simulink model "Circuito"  (R2014a)
settings: Solver=ode45  StartTime=0.0  StopTime=100  RelTol=1e-3
PreLoadFcn:
  | variables
InitFcn:
  | eval('variables');
  | variables
StartFcn:
  | variables
libraries: fl_lib x44, nesl_utility x5
settings Model: Creator=jhoan  LastModifiedBy=jhoan

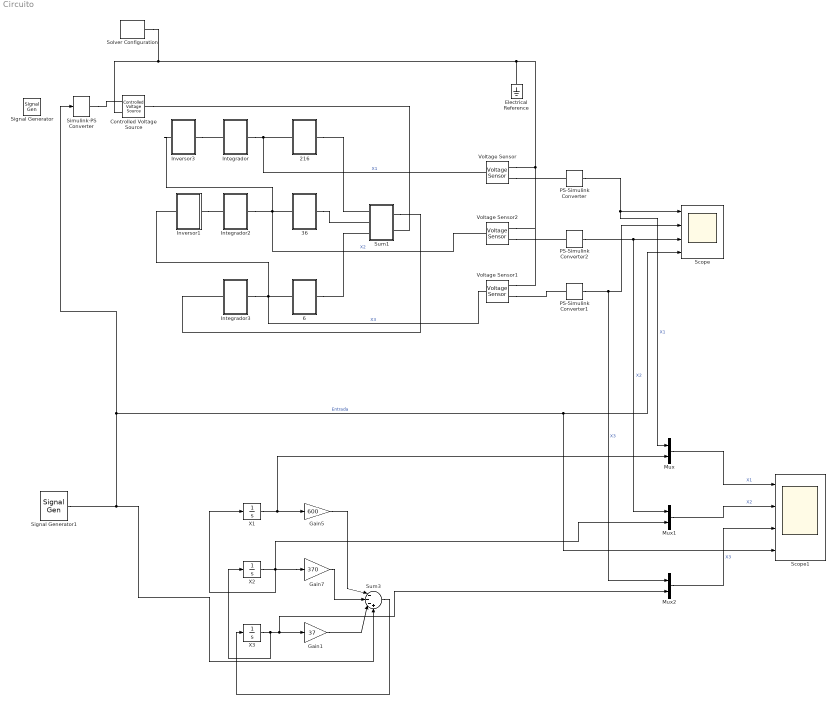
== system Circuito ==
  216 : Subsystem
  36 : Subsystem
  6 : Subsystem
  Controlled Voltage Source : fl_lib/Electrical/Electrical Sources/Controlled Voltage Source
  Electrical Reference : fl_lib/Electrical/Electrical Elements/Electrical Reference
  Gain1 : Gain  Gain=37
  Gain5 : Gain  Gain=600
  Gain7 : Gain  Gain=370
  Integrador : Subsystem
  Integrador2 : Subsystem
  Integrador3 : Subsystem
  Inversor1 : Subsystem
  Inversor3 : Subsystem
  Mux : Mux  Inputs=2
  Mux1 : Mux  Inputs=2
  Mux2 : Mux  Inputs=2
  PS-Simulink Converter : nesl_utility/PS-Simulink Converter  PhysicalDomain=network_engine_domain  SubClassName=ps_output  LeftPortType=input  RightPortType=output  PseudoPeriodic=off  Frequencies=[]  Unit=1  AffineConversion=off
  PS-Simulink Converter1 : nesl_utility/PS-Simulink Converter  PhysicalDomain=network_engine_domain  SubClassName=ps_output  LeftPortType=input  RightPortType=output  PseudoPeriodic=off  Frequencies=[]  Unit=1  AffineConversion=off
  PS-Simulink Converter2 : nesl_utility/PS-Simulink Converter  PhysicalDomain=network_engine_domain  SubClassName=ps_output  LeftPortType=input  RightPortType=output  PseudoPeriodic=off  Frequencies=[]  Unit=1  AffineConversion=off
  Scope : Scope  NumInputPorts=4
      settings: YMin=-5~-5~-5~-5  YMax=5~5~5~5
  Scope1 : Scope  NumInputPorts=4
      settings: TimeRange=0.323900041697037  YMin=-5~-5~0.09553514947454364~-5  YMax=5~5~0.09836343230282654~5  SaveName=subSimulink
  Signal Generator : SignalGenerator  Amplitude=2  Frequency=10
  Signal Generator1 : SignalGenerator  WaveForm=square  Amplitude=2  Frequency=0.1
  Simulink-PS Converter : nesl_utility/Simulink-PS Converter  PhysicalDomain=network_engine_domain  SubClassName=ps_input  LeftPortType=input  RightPortType=output  PseudoPeriodic=off  Frequencies=[]  NoiseDistribution=none  NoiseParameters=[]  Unit=1  AffineConversion=off  InputFiltering=off  SimscapeFilterOrder=1  InputFilterTimeConstant=0.001  UdotUserProvided=1
  Solver Configuration : nesl_utility/Solver Configuration  PhysicalDomain=network_engine_domain  SubClassName=solver  LeftPortType=input  RightPortType=generic  Accelerate=off  Tones=[]  Harmonics=[]  SimulateNoise=off  Profile=off  UseLocalSampling=off  EnableSwitchedLinearOptims=on  FrequencyDomain=off  UseCCode=off  RelTol=0.001  AbsTol=1e-06  MinStep=1e-09  ToWorkspace=off  DoDC=off  ResidualTolerance=1e-09  UseLocalSolver=off  LocalSolverChoice=NE_BACKWARD_EULER_ADVANCER  LocalSolverSampleTime=0.001  DoFixedCost=off  MaxNonlinIter=3  MaxModeIter=2  LinearAlgebra=Sparse  DelaysMemoryBudget=1024  AutomaticFiltering=on  FilteringTimeConstant=0.001
  Sum1 : Subsystem
  Sum3 : Sum  Inputs=|---+
  Voltage Sensor : fl_lib/Electrical/Electrical Sensors/Voltage Sensor
  Voltage Sensor1 : fl_lib/Electrical/Electrical Sensors/Voltage Sensor
  Voltage Sensor2 : fl_lib/Electrical/Electrical Sensors/Voltage Sensor
  X1 : Integrator
  X2 : Integrator
  "X3 " : Integrator
  wires:
  PS-Simulink Converter/1 -> Mux/1, Scope/1  "X1"
  PS-Simulink Converter1/1 -> Mux2/1, Scope/2  "X3"
  PS-Simulink Converter2/1 -> Mux1/1, Scope/3  "X2"
  "X3 "/1 -> X2/1, Mux2/2, Gain1/1
  Gain5/1 -> Sum3/1
  Gain7/1 -> Sum3/2
  Gain1/1 -> Sum3/3
  Signal Generator1/1 -> Scope1/4, Scope/4, Simulink-PS Converter/1, Sum3/4  "Entrada"
  Sum3/1 -> "X3 "/1
  X1/1 -> Mux/2, Gain5/1
  Mux/1 -> Scope1/1  "X1"
  X2/1 -> X1/1, Gain7/1, Mux1/2
  Mux2/1 -> Scope1/3  "X3"
  Mux1/1 -> Scope1/2  "X2"
  connections:
  Solver Configuration/RConn1 -- Controlled Voltage Source/RConn2 -- Voltage Sensor2/RConn2 -- Voltage Sensor1/RConn2 -- Voltage Sensor/RConn2 -- Electrical Reference/LConn1
  Voltage Sensor/RConn1 -- PS-Simulink Converter/LConn1
  Simulink-PS Converter/RConn1 -- Controlled Voltage Source/RConn1
  Voltage Sensor1/RConn1 -- PS-Simulink Converter1/LConn1
  Integrador/RConn1 -- Voltage Sensor/LConn1 -- 216/LConn1  "X1"
  Integrador3/RConn1 -- Inversor1/LConn1 -- Voltage Sensor1/LConn1 -- 6/LConn1  "X3"
  216/RConn1 -- Sum1/LConn1
  36/RConn1 -- Sum1/LConn2
  6/RConn1 -- Sum1/LConn3
  Controlled Voltage Source/LConn1 -- Sum1/RConn2
  Integrador2/RConn1 -- Voltage Sensor2/LConn1 -- Inversor3/LConn1 -- 36/LConn1  "X2"
  Voltage Sensor2/RConn1 -- PS-Simulink Converter2/LConn1
  Inversor3/RConn1 -- Integrador/LConn1
  Inversor1/RConn1 -- Integrador2/LConn1
  Sum1/RConn1 -- Integrador3/LConn1

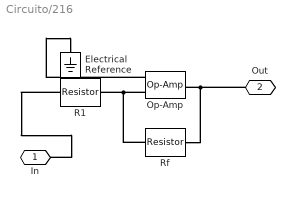
== system Circuito/216 ==
  Electrical Reference : fl_lib/Electrical/Electrical Elements/Electrical Reference
  Op-Amp : fl_lib/Electrical/Electrical Elements/Op-Amp  outI_specify=off  outI_priority=High  outI=0 A
  R1 : fl_lib/Electrical/Electrical Elements/Resistor  R=1 Ohm  i_specify=off  i_priority=High  i=0 A  v_specify=off  v_priority=High  v=0 V
  Rf : fl_lib/Electrical/Electrical Elements/Resistor  R=600 Ohm  i_specify=off  i_priority=High  i=0 A  v_specify=off  v_priority=High  v=0 V
  In : PMIOPort  Port=1  Side=Left
  Out : PMIOPort  Port=2  Side=Right
  connections:
  R1/LConn1 -- In/RConn1
  Out/RConn1 -- Rf/RConn1 -- Op-Amp/RConn1
  Op-Amp/LConn1 -- Electrical Reference/LConn1
  Op-Amp/LConn2 -- Rf/LConn1 -- R1/RConn1

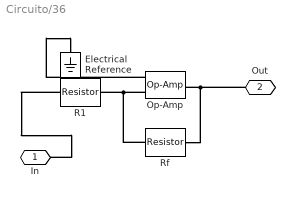
== system Circuito/36 ==
  Electrical Reference : fl_lib/Electrical/Electrical Elements/Electrical Reference
  Op-Amp : fl_lib/Electrical/Electrical Elements/Op-Amp  outI_specify=off  outI_priority=High  outI=0 A
  R1 : fl_lib/Electrical/Electrical Elements/Resistor  R=1 Ohm  i_specify=off  i_priority=High  i=0 A  v_specify=off  v_priority=High  v=0 V
  Rf : fl_lib/Electrical/Electrical Elements/Resistor  R=370 Ohm  i_specify=off  i_priority=High  i=0 A  v_specify=off  v_priority=High  v=0 V
  In : PMIOPort  Port=1  Side=Left
  Out : PMIOPort  Port=2  Side=Right
  connections:
  R1/LConn1 -- In/RConn1
  Out/RConn1 -- Rf/RConn1 -- Op-Amp/RConn1
  Op-Amp/LConn1 -- Electrical Reference/LConn1
  Op-Amp/LConn2 -- Rf/LConn1 -- R1/RConn1

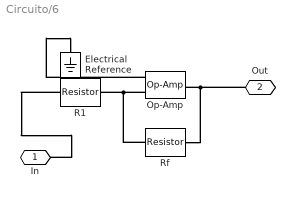
== system Circuito/6 ==
  Electrical Reference : fl_lib/Electrical/Electrical Elements/Electrical Reference
  Op-Amp : fl_lib/Electrical/Electrical Elements/Op-Amp  outI_specify=off  outI_priority=High  outI=0 A
  R1 : fl_lib/Electrical/Electrical Elements/Resistor  R=1 Ohm  i_specify=off  i_priority=High  i=0 A  v_specify=off  v_priority=High  v=0 V
  Rf : fl_lib/Electrical/Electrical Elements/Resistor  R=37 Ohm  i_specify=off  i_priority=High  i=0 A  v_specify=off  v_priority=High  v=0 V
  In : PMIOPort  Port=1  Side=Left
  Out : PMIOPort  Port=2  Side=Right
  connections:
  R1/LConn1 -- In/RConn1
  Out/RConn1 -- Rf/RConn1 -- Op-Amp/RConn1
  Op-Amp/LConn1 -- Electrical Reference/LConn1
  Op-Amp/LConn2 -- Rf/LConn1 -- R1/RConn1

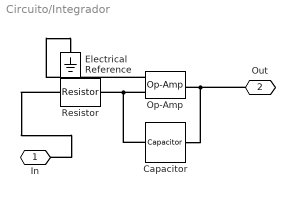
== system Circuito/Integrador ==
  Capacitor : fl_lib/Electrical/Electrical Elements/Capacitor  c=1e-6 F  r=1e-6 Ohm  g=0 1/Ohm  i_specify=off  i_priority=High  i=0 A  v_specify=off  v_priority=High  v=0 V  vc_specify=off  vc_priority=High  vc=0 V
  Electrical Reference : fl_lib/Electrical/Electrical Elements/Electrical Reference
  Op-Amp : fl_lib/Electrical/Electrical Elements/Op-Amp  outI_specify=off  outI_priority=High  outI=0 A
  Resistor : fl_lib/Electrical/Electrical Elements/Resistor  R=1 MOhm  i_specify=off  i_priority=High  i=0 A  v_specify=off  v_priority=High  v=0 V
  In : PMIOPort  Port=1  Side=Left
  Out : PMIOPort  Port=2  Side=Right
  connections:
  Resistor/LConn1 -- In/RConn1
  Capacitor/RConn1 -- Out/RConn1 -- Op-Amp/RConn1
  Op-Amp/LConn1 -- Electrical Reference/LConn1
  Op-Amp/LConn2 -- Capacitor/LConn1 -- Resistor/RConn1

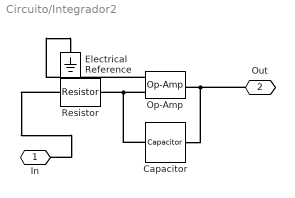
== system Circuito/Integrador2 ==
  Capacitor : fl_lib/Electrical/Electrical Elements/Capacitor  c=1e-6 F  r=1e-6 Ohm  g=0 1/Ohm  i_specify=off  i_priority=High  i=0 A  v_specify=off  v_priority=High  v=0 V  vc_specify=off  vc_priority=High  vc=0 V
  Electrical Reference : fl_lib/Electrical/Electrical Elements/Electrical Reference
  Op-Amp : fl_lib/Electrical/Electrical Elements/Op-Amp  outI_specify=off  outI_priority=High  outI=0 A
  Resistor : fl_lib/Electrical/Electrical Elements/Resistor  R=1 MOhm  i_specify=off  i_priority=High  i=0 A  v_specify=off  v_priority=High  v=0 V
  In : PMIOPort  Port=1  Side=Left
  Out : PMIOPort  Port=2  Side=Right
  connections:
  Resistor/LConn1 -- In/RConn1
  Capacitor/RConn1 -- Out/RConn1 -- Op-Amp/RConn1
  Op-Amp/LConn1 -- Electrical Reference/LConn1
  Op-Amp/LConn2 -- Capacitor/LConn1 -- Resistor/RConn1

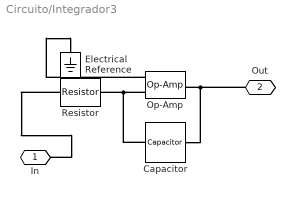
== system Circuito/Integrador3 ==
  Capacitor : fl_lib/Electrical/Electrical Elements/Capacitor  c=1e-6 F  r=1e-6 Ohm  g=0 1/Ohm  i_specify=off  i_priority=High  i=0 A  v_specify=off  v_priority=High  v=0 V  vc_specify=off  vc_priority=High  vc=0 V
  Electrical Reference : fl_lib/Electrical/Electrical Elements/Electrical Reference
  Op-Amp : fl_lib/Electrical/Electrical Elements/Op-Amp  outI_specify=off  outI_priority=High  outI=0 A
  Resistor : fl_lib/Electrical/Electrical Elements/Resistor  R=1 MOhm  i_specify=off  i_priority=High  i=0 A  v_specify=off  v_priority=High  v=0 V
  In : PMIOPort  Port=1  Side=Left
  Out : PMIOPort  Port=2  Side=Right
  connections:
  Resistor/LConn1 -- In/RConn1
  Capacitor/RConn1 -- Out/RConn1 -- Op-Amp/RConn1
  Op-Amp/LConn1 -- Electrical Reference/LConn1
  Op-Amp/LConn2 -- Capacitor/LConn1 -- Resistor/RConn1

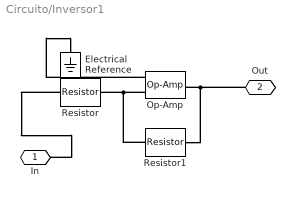
== system Circuito/Inversor1 ==
  Electrical Reference : fl_lib/Electrical/Electrical Elements/Electrical Reference
  Op-Amp : fl_lib/Electrical/Electrical Elements/Op-Amp  outI_specify=off  outI_priority=High  outI=0 A
  Resistor : fl_lib/Electrical/Electrical Elements/Resistor  R=1 kOhm  i_specify=off  i_priority=High  i=0 A  v_specify=off  v_priority=High  v=0 V
  Resistor1 : fl_lib/Electrical/Electrical Elements/Resistor  R=1 kOhm  i_specify=off  i_priority=High  i=0 A  v_specify=off  v_priority=High  v=0 V
  In : PMIOPort  Port=1  Side=Left
  Out : PMIOPort  Port=2  Side=Right
  connections:
  Resistor/LConn1 -- In/RConn1
  Out/RConn1 -- Resistor1/RConn1 -- Op-Amp/RConn1
  Op-Amp/LConn1 -- Electrical Reference/LConn1
  Op-Amp/LConn2 -- Resistor1/LConn1 -- Resistor/RConn1

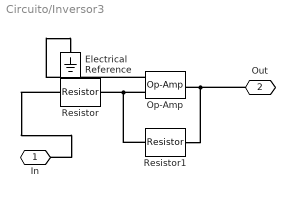
== system Circuito/Inversor3 ==
  Electrical Reference : fl_lib/Electrical/Electrical Elements/Electrical Reference
  Op-Amp : fl_lib/Electrical/Electrical Elements/Op-Amp  outI_specify=off  outI_priority=High  outI=0 A
  Resistor : fl_lib/Electrical/Electrical Elements/Resistor  R=1 kOhm  i_specify=off  i_priority=High  i=0 A  v_specify=off  v_priority=High  v=0 V
  Resistor1 : fl_lib/Electrical/Electrical Elements/Resistor  R=1 kOhm  i_specify=off  i_priority=High  i=0 A  v_specify=off  v_priority=High  v=0 V
  In : PMIOPort  Port=1  Side=Left
  Out : PMIOPort  Port=2  Side=Right
  connections:
  Resistor/LConn1 -- In/RConn1
  Out/RConn1 -- Resistor1/RConn1 -- Op-Amp/RConn1
  Op-Amp/LConn1 -- Electrical Reference/LConn1
  Op-Amp/LConn2 -- Resistor1/LConn1 -- Resistor/RConn1

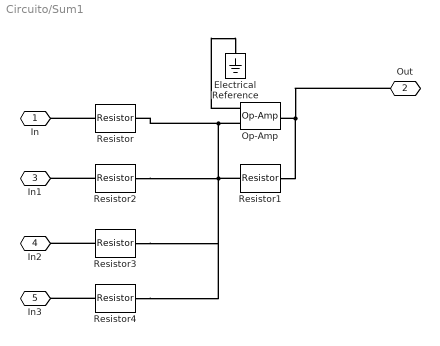
== system Circuito/Sum1 ==
  Electrical Reference : fl_lib/Electrical/Electrical Elements/Electrical Reference
  Op-Amp : fl_lib/Electrical/Electrical Elements/Op-Amp  outI_specify=off  outI_priority=High  outI=0 A
  Resistor{,1..4} (5 alike) : fl_lib/Electrical/Electrical Elements/Resistor  R=1 kOhm  i_specify=off  i_priority=High  i=0 A  v_specify=off  v_priority=High  v=0 V
  In : PMIOPort  Port=1  Side=Left
  Out : PMIOPort  Port=2  Side=Right
  In1 : PMIOPort  Port=3  Side=Left
  In2 : PMIOPort  Port=4  Side=Right
  In3 : PMIOPort  Port=5  Side=Left
  connections:
  Resistor/LConn1 -- In/RConn1
  Out/RConn1 -- Op-Amp/RConn1 -- Resistor1/RConn1
  Op-Amp/LConn1 -- Electrical Reference/LConn1
  Op-Amp/LConn2 -- Resistor1/LConn1 -- Resistor4/RConn1 -- Resistor3/RConn1 -- Resistor2/RConn1 -- Resistor/RConn1
  Resistor2/LConn1 -- In1/RConn1
  Resistor3/LConn1 -- In2/RConn1
  Resistor4/LConn1 -- In3/RConn1
